simulink model "ros2_symulink_ettorone_mujoco"  (R2025b)
settings: Solver=ode4  StartTime=0.0  StopTime=inf  FixedStep=0.002  RelTol=1e-3
libraries: slpidlib x12, ros2lib x5
settings Model: Creator=ema  LastModifiedBy=ema

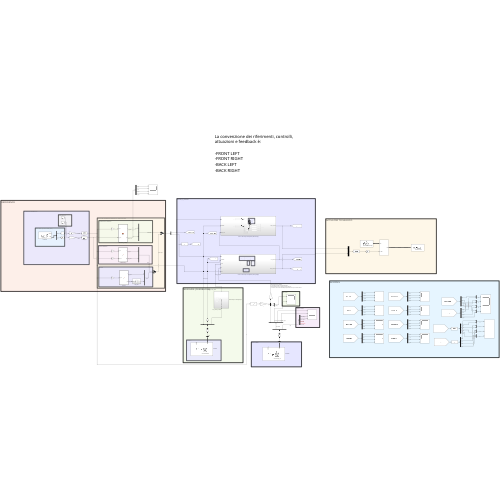
[thumbnail: Simulink's stored preview of the top-level diagram]
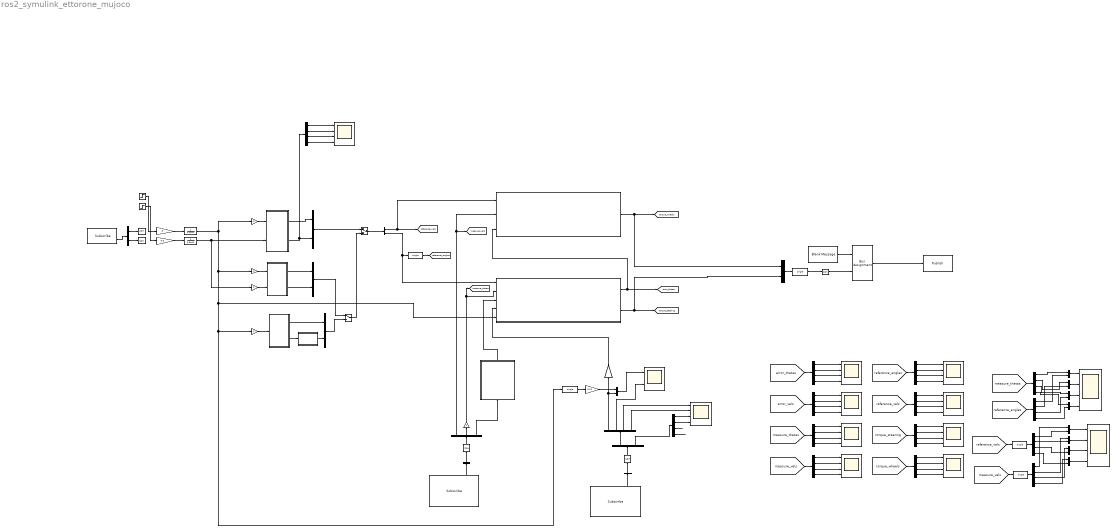
== system ros2_symulink_ettorone_mujoco ==
  note: La convenzione dei riferimenti, controlli, attuazioni e feedback è:
      |
      | -FRONT LEFT
      | -FRONT RIGHT
      | -BACK LEFT
      | -BACK RIGHT
  note: WHEELS SLIPS
  note: body_twist
  note: BODY FRAME
  note: WHEELS
  note: LOW LEVEL REFERENCE GENERATOR / MODE CONTROL
  note: SPIN360
  note: ROS2 INPUT (JOYSTIC CMD_VEL)
  note: const reference
  note: SCOPES
  note: MOTORS_&_CONTROL
  note: MEASURE (FEEDBACKS)
  note: ACTUATOR TO MUJOCO
  note: REFERENCE
  note: REFERENCE GENERATOR
  note: ACKERMANN STEERING
  note: CRAB STEERING
  Blank Message : ros2lib/Blank Message  messageClass=Message  entityType=interfaces/Float32Array8  messageType=interfaces/Float32Array8  SampleTime=0.002
  Bus Assignment : BusAssignment  AssignedSignals=data
  Bus Selector : BusSelector  OutputSignals=data
  Bus Selector1 : BusSelector  OutputSignals=linear.x,angular.z
  Bus Selector2 : BusSelector  OutputSignals=data
  Crab steering : MATLAB Function  TreatAsAtomicUnit=on
  Data Type Conversion{1..5} (5 alike) : DataTypeConversion  OutDataTypeStr=single  SaturateOnIntegerOverflow=off  RndMeth=Floor
  Demux1 : Demux  Outputs=3
  Demux{2..4,6..13,16..19} (15 alike) : Demux
  Demux15 : Demux  Outputs=2
  Demux5 : Demux  Outputs=2
  Gain : Gain
  Gain1 : Gain  Gain=8
  Gain2 : Gain  Gain=0.5
  Gain3 : Gain  Gain=1/0.12
  Gain5 : Gain  Gain=-1
  Gain6 : Gain
  Gain7 : Gain  Gain=-1
  Gain8 : Gain  Gain=-1
  Manual Switch : ManualSwitch
  Manual Switch1 : ManualSwitch
  Mux{,1..7,9..13} (13 alike) : Mux  Inputs=2
  Publish : ros2lib/Publish  topicSource=Specify your own  topic=/ettorone/actuator  messageType=interfaces/Float32Array8  QOSHistory=Keep last  QOSDepth=10  QOSReliability=Reliable  QOSDurability=Volatile  QOSDeadline=Inf  QOSLifespan=Inf  QOSLiveliness=Automatic  QOSLeaseDuration=Inf  QOSAvoidROSNamespaceConventions=off
  Scope{1..10,12..13} (12 alike) : Scope  NumInputPorts=4
      Scope1 settings: ActiveDisplayYMinimum=-24.08971523267201  ActiveDisplayYMaximum=2.6766350258524776
      Scope10 settings: ActiveDisplayString=4  ActiveDisplayYMinimum=-0.352103733781405  ActiveDisplayYMaximum=0.039646837980399134  DataLoggingVariableName=ScopeData10
      Scope12 settings: ActiveDisplayString=4  ActiveDisplayYMinimum=-12.276754975318909  ActiveDisplayYMaximum=1.3640838861465452  DataLoggingVariableName=ScopeData13
      Scope13 settings: ActiveDisplayYMinimum=-0.22020444087684155  ActiveDisplayYMaximum=0.25354055874049664  DataLoggingVariableName=ScopeData12
      Scope2 settings: ActiveDisplayYMinimum=-24.08971523267201  ActiveDisplayYMaximum=2.6766350258524776  DataLoggingVariableName=ScopeData3
      Scope3 settings: ActiveDisplayYMinimum=-24.08971523267201  ActiveDisplayYMaximum=2.6766350258524776
      Scope4 settings: ActiveDisplayYMinimum=-24.08971523267201  ActiveDisplayYMaximum=2.6766350258524776  DataLoggingVariableName=ScopeData2
      Scope5 settings: ActiveDisplayYMinimum=-24.08971523267201  ActiveDisplayYMaximum=2.6766350258524776  DataLoggingVariableName=ScopeData4
      Scope6 settings: ActiveDisplayYMinimum=-24.08971523267201  ActiveDisplayYMaximum=2.6766350258524776  DataLoggingVariableName=ScopeData5
      Scope7 settings: ActiveDisplayYMinimum=-24.08971523267201  ActiveDisplayYMaximum=2.6766350258524776  DataLoggingVariableName=ScopeData6
      Scope8 settings: ActiveDisplayYMinimum=-24.08971523267201  ActiveDisplayYMaximum=2.6766350258524776  DataLoggingVariableName=ScopeData7
      Scope9 settings: ActiveDisplayYMinimum=-0.038596316224778507  ActiveDisplayYMaximum=0.3473668460230066  DataLoggingVariableName=ScopeData8
  Scope11 : Scope  NumInputPorts=2
      settings: ActiveDisplayYMinimum=-0.10174171955077324  ActiveDisplayYMaximum=0.915423120426567  DataLoggingVariableName=ScopeData11
  Step : Step  Time=0  SampleTime=0
  Step1 : Step  Time=10  After=0.5  SampleTime=0
  Wheel Torque to Steering Torque : Subsystem
  Zero-Order Hold{,1..4} (5 alike) : ZeroOrderHold  SampleTime=0.002
  ackermann_geometry : MATLAB Function  TreatAsAtomicUnit=on
  control + motor torque linear dynamic (steering angles) : Subsystem
  control + motor torque linear dynamic (wheel velocity) : Subsystem
  feedback : ros2lib/Subscribe  topicSource=Specify your own  topic=/ettorone/feedback  messageType=interfaces/Float32Array12  sampleTime=0.002  QOSHistory=Keep last  QOSDepth=10  QOSReliability=Best effort  QOSDurability=Volatile  QOSDeadline=Inf  QOSLifespan=Inf  QOSLiveliness=Automatic  QOSLeaseDuration=Inf  QOSAvoidROSNamespaceConventions=off
  feedback1 : ros2lib/Subscribe  topicSource=Specify your own  topic=/joy/cmd_vel  messageType=geometry_msgs/Twist  sampleTime=0.002  QOSHistory=Keep last  QOSDepth=10  QOSReliability=Best effort  QOSDurability=Volatile  QOSDeadline=Inf  QOSLifespan=Inf  QOSLiveliness=Automatic  QOSLeaseDuration=Inf  QOSAvoidROSNamespaceConventions=off
  feedback2 : ros2lib/Subscribe  topicSource=Specify your own  topic=/ettorone/body_vel  messageType=interfaces/Float32Array8  sampleTime=0.002  QOSHistory=Keep last  QOSDepth=10  QOSReliability=Best effort  QOSDurability=Volatile  QOSDeadline=Inf  QOSLifespan=Inf  QOSLiveliness=Automatic  QOSLeaseDuration=Inf  QOSAvoidROSNamespaceConventions=off
  filters_a : TransferFcn  Denominator=[0.5 1]
  filters_v : TransferFcn  Denominator=[0.1 1]
  r : Gain  Gain=0.12
  spin mod : MATLAB Function  TreatAsAtomicUnit=on
  spin_filters : Subsystem
  tag scope: error_thetas=global, measure_thetas=global, measure_vels=global, reference_angles=global, reference_vels=global, torque_steering=global, torque_wheels=global
  wires:
  Blank Message/1 -> Bus Assignment/1
  Bus Assignment/1 -> Publish/1
  Zero-Order Hold/1 -> Demux1/1
  control + motor torque linear dynamic (wheel velocity)/1(Torque_wheels) -> [torque_wheels], Mux/1
  Demux1/1 -> control + motor torque linear dynamic (wheel velocity)/2(feedback), [measure_vels]  "wheels_vels"
  Demux1/2 -> Gain/1
  feedback/2 -> Bus Selector/1
  Bus Selector/1 -> Zero-Order Hold/1  "<data>"
  Zero-Order Hold2/1 -> Bus Assignment/2
  Mux/1 -> Data Type Conversion1/1
  Data Type Conversion1/1 -> Zero-Order Hold2/1
  Gain/1 -> [measure_thetas], control + motor torque linear dynamic (steering angles)/2(feedback)  "wheels_steering_angles"
  control + motor torque linear dynamic (steering angles)/2(Torque_steering) -> [torque_steering], Mux/2
  Bus Selector1/1 -> Zero-Order Hold1/1  "<x>"
  feedback1/2 -> Bus Selector1/1
  Bus Selector1/2 -> Zero-Order Hold3/1  "<z>"
  Crab steering/1(v) -> Mux3/1  "v_k_des"
  Crab steering/2(phi) -> Mux3/2  "phi_k_des"
  ackermann_geometry/2(phi) -> Demux11/1, Mux1/2  "phi_k_des"
  Manual Switch/1 -> Demux5/1
  Mux1/1 -> Manual Switch/1  "ackermann"
  ackermann_geometry/1(v) -> Mux1/1  "v_k_des"
  Demux5/1 -> [reference_vels], control + motor torque linear dynamic (wheel velocity)/1(ref)
  filters_a/1 -> ackermann_geometry/2(phi_des), Gain6/1
  Gain5/1 -> Crab steering/1(v_des)
  Gain6/1 -> Crab steering/2(phi_des)
  Gain7/1 -> ackermann_geometry/1(v_des)
  Demux1/3 -> Wheel Torque to Steering Torque/1(torque_whhels_feedback)  "torque_wheels_feedback"
  Wheel Torque to Steering Torque/1(Out1) -> control + motor torque linear dynamic (steering angles)/3(torch)  "torque_projected"
  control + motor torque linear dynamic (steering angles)/1(error_steering) -> [error_thetas], control + motor torque linear dynamic (wheel velocity)/3(theta_error)
  [error_thetas] -> Demux2/1
  [error_vels] -> Demux3/1
  Demux2/1 -> Scope6/1  "e_th_fl"
  Demux2/2 -> Scope6/2  "e_th_fr"
  Demux2/3 -> Scope6/3  "e_th_bl"
  Demux2/4 -> Scope6/4  "e_th_br"
  Demux3/1 -> Scope5/1  "e_v_fl"
  Demux3/2 -> Scope5/2  "e_v_fr"
  Demux3/3 -> Scope5/3  "e_v_bl"
  Demux3/4 -> Scope5/4  "e_v_br"
  Demux4/2 -> Scope2/2  "th_fr"
  Demux6/4 -> Scope1/4  "v_br"
  Demux6/2 -> Scope1/2  "v_fr"
  [measure_thetas] -> Demux4/1
  Demux6/3 -> Scope1/3  "v_bl"
  [measure_vels] -> Demux6/1
  Demux4/1 -> Scope2/1  "th_fl"
  Demux6/1 -> Scope1/1  "v_fl"
  Demux4/3 -> Scope2/3  "th_bl"
  Demux4/4 -> Scope2/4  "th_br"
  Demux7/2 -> Scope3/2  "r_th_fr"
  Demux8/4 -> Scope4/4  "r_v_br"
  Demux8/2 -> Scope4/2  "r_v_fr"
  [reference_angles] -> Demux7/1
  Demux8/3 -> Scope4/3  "r_v_bl"
  [reference_vels] -> Demux8/1
  Demux7/1 -> Scope3/1  "r_th_fl"
  Demux8/1 -> Scope4/1  "r_v_fl"
  Demux7/3 -> Scope3/3  "r_th_bl"
  Demux7/4 -> Scope3/4  "r_th_br"
  Demux9/4 -> Scope7/4  "t_th_br"
  [torque_steering] -> Demux9/1
  [torque_wheels] -> Demux10/1
  Demux10/4 -> Scope8/4  "t_v_br"
  Demux10/2 -> Scope8/2  "t_v_fr"
  Demux10/3 -> Scope8/3  "t_v_bl"
  Demux9/3 -> Scope7/3  "t_th_bl"
  Demux9/1 -> Scope7/1  "t_th_fl"
  Demux10/1 -> Scope8/1  "t_v_fl"
  Demux9/2 -> Scope7/2  "t_th_fr"
  Demux11/4 -> Scope9/4  "r_th_br"
  Demux11/3 -> Scope9/3  "r_th_bl"
  Demux11/1 -> Scope9/1  "r_th_fl"
  Demux11/2 -> Scope9/2  "r_th_fr"
  [reference_angles] -> Demux13/1
  Mux2/1 -> Scope10/1  "fl"
  Mux4/1 -> Scope10/2  "fr"
  Mux5/1 -> Scope10/3  "bl"
  Demux13/1 -> Mux2/2  "r_th_fl"
  Demux13/2 -> Mux4/2  "r_th_fr"
  Demux13/3 -> Mux5/2  "r_th_bl"
  Demux13/4 -> Mux6/2  "r_th_br"
  Mux6/1 -> Scope10/4  "br"
  Demux12/2 -> Mux4/1  "v_fr"
  [measure_thetas] -> Demux12/1
  Demux12/3 -> Mux5/1  "v_bl"
  Demux12/1 -> Mux2/1  "v_fl"
  Demux12/4 -> Mux6/1  "v_br"
  Data Type Conversion2/1 -> [reference_angles]
  Demux5/2 -> control + motor torque linear dynamic (steering angles)/1(ref), Data Type Conversion2/1
  spin mod/1(v) -> Mux7/1  "v_k_des"
  Mux3/1 -> Manual Switch1/1  "grab"
  Mux7/1 -> Manual Switch1/2  "spin"
  Manual Switch1/1 -> Manual Switch/2  "grab or spin"
  feedback2/2 -> Bus Selector2/1
  Zero-Order Hold4/1 -> Demux15/1
  Bus Selector2/1 -> Zero-Order Hold4/1  "<data>"
  Demux16/2 -> Scope11/2  "yaw_rate"
  Demux16/1 -> Gain3/1, Mux13/2  "vx"
  Demux15/1 -> Demux16/1  "vels & slips"
  Gain1/1 -> filters_v/1  "velocities"
  Gain2/1 -> filters_a/1  "angles"
  Gain3/1 -> control + motor torque linear dynamic (steering angles)/4(vx)  "volendo questo si puo cambiare è un termine che prende la velocità longitudinale nel body frame del rover è lo divide per il raggio delle ruote. cosi da avere due velocità confrontabili per il gain dinamico del FF per il sistema di sterzo"
  [reference_vels] -> Data Type Conversion5/1
  Mux12/1 -> Scope12/4  "br"
  Mux10/1 -> Scope12/2  "fr"
  Mux11/1 -> Scope12/3  "bl"
  Mux9/1 -> Scope12/1  "fl"
  [measure_vels] -> Data Type Conversion4/1
  Mux13/1 -> Scope11/1  "v_long"
  Data Type Conversion3/1 -> r/1
  Data Type Conversion4/1 -> Demux18/1
  Data Type Conversion5/1 -> Demux17/1
  Demux15/2 -> Demux19/1  "slip"
  Demux16/3 -> Scope13/1  "angle_slip_fl"
  Demux16/4 -> Scope13/2  "angle_slip_fr"
  Demux19/1 -> Scope13/3  "angle_slip_bl"
  Demux19/2 -> Scope13/4  "angle_slip_br"
  filters_v/1 -> Data Type Conversion3/1, Gain8/1, control + motor torque linear dynamic (steering angles)/5(vref), Gain5/1, Gain7/1  "w"
  r/1 -> Mux13/1  "v_long_ref"
  Demux17/1 -> Mux9/2  "r_v_fl"
  Demux17/2 -> Mux10/2  "r_v_fr"
  Demux17/3 -> Mux11/2  "r_v_bl"
  Demux17/4 -> Mux12/2  "r_v_br"
  Demux18/1 -> Mux9/1  "v_fl"
  Demux18/2 -> Mux10/1  "v_fr"
  Demux18/3 -> Mux11/1  "v_bl"
  Demux18/4 -> Mux12/1  "v_br"
  Step/1 -> Gain1/1  "rotational speed ref"
  Step1/1 -> Gain2/1
  Gain8/1 -> spin mod/1(v_des)
  spin mod/2(phi) -> spin_filters/1(phi_k_des)  "phi_k_des"
  spin_filters/1(Out1) -> Mux7/2
  Demux19/3 -> ?  "non usato"
  Demux19/4 -> ?  "non usato"

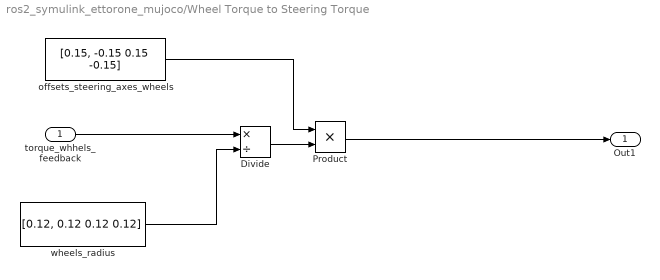
== system ros2_symulink_ettorone_mujoco/Wheel Torque to Steering Torque ==
  torque_whhels_feedback : Inport
  Divide : Product  Inputs=*/
  Product : Product
  offsets_steering_axes_wheels : Constant  Value=[0.15, -0.15 0.15 -0.15]
  wheels_radius : Constant  Value=[0.12, 0.12 0.12 0.12]
  Out1 : Outport
  wires:
  wheels_radius/1 -> Divide/2
  Divide/1 -> Product/2
  offsets_steering_axes_wheels/1 -> Product/1
  torque_whhels_feedback/1 -> Divide/1
  Product/1 -> Out1/1

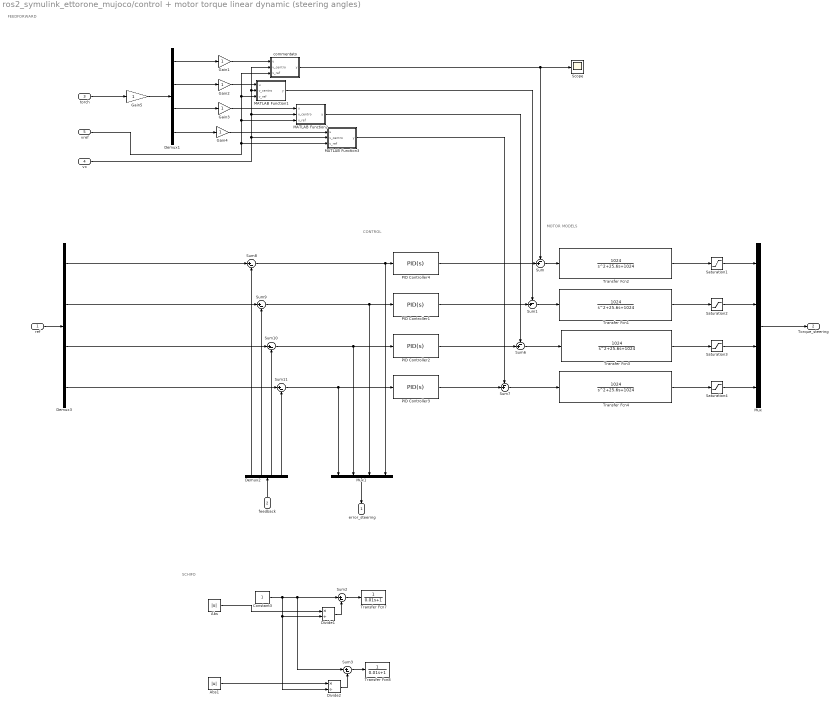
== system ros2_symulink_ettorone_mujoco/control + motor torque linear dynamic (steering angles) ==
  note: SCHIFO
  note: MOTOR MODELS
  note: CONTROL
  note: FEEDFORWARD
  ref : Inport
  feedback : Inport  Port=2
  torch : Inport  Port=3
  vx : Inport  Port=4
  vref : Inport  Port=5
  Abs : Abs  SaturateOnIntegerOverflow=off
  Abs1 : Abs  SaturateOnIntegerOverflow=off
  Constant3 : Constant
  Demux1 : Demux
  Demux2 : Demux
  Demux3 : Demux
  Divide1 : Product  Inputs=*/
  Divide2 : Product  Inputs=*/
  Gain{1..5} (5 alike) : Gain
  MATLAB Function1 : MATLAB Function  TreatAsAtomicUnit=on
  MATLAB Function2 : MATLAB Function  TreatAsAtomicUnit=on
  MATLAB Function3 : MATLAB Function  TreatAsAtomicUnit=on
  Mux : Mux
  Mux1 : Mux
  PID Controller1 : slpidlib/PID Controller  Controller=PID  Form=Parallel  TimeDomain=Continuous-time  UseExternalTs=off  SampleTime=-1  IntegratorMethod=Forward Euler  FilterMethod=Forward Euler  ControllerParametersSource=internal  P=30  I=4  UseKiTs=off  D=0  UseExternalDerivativeSource=off  N=100  UseFilter=on  TunerSelectOption=Transfer Function Based (PID Tuner App)  InitialConditionSource=internal  InitialConditionForIntegrator=0  InitialConditionForFilter=0  DifferentiatorICPrevScaledInput=0  ExternalReset=none  TrackingMode=off  Kt=1  LimitOutput=on  SatLimitsSource=internal  UpperSaturationLimit=25  LowerSaturationLimit=-25  LinearizeAsGain=on  AntiWindupMode=back-calculation  Kb=1  LimitIntegrator=off  UpperIntegratorSaturationLimit=inf  LowerIntegratorSaturationLimit=-inf  POutMin=[]  POutMax=[]  IOutMin=[]  IOutMax=[]  DOutMin=[]  DOutMax=[]  NOutMin=[]  NOutMax=[]  SumOutMin=[]  SumOutMax=[]  SaturationOutMin=[]  SaturationOutMax=[]  PParamMin=[]  PParamMax=[]  IParamMin=[]  IParamMax=[]  DParamMin=[]  DParamMax=[]  NParamMin=[]  NParamMax=[]  KbParamMin=[]  KbParamMax=[]  KtParamMin=[]  KtParamMax=[]  KbOutMin=[]  KbOutMax=[]  KtOutMin=[]  KtOutMax=[]  IntegratorOutMin=[]  IntegratorOutMax=[]  FilterOutMin=[]  FilterOutMax=[]  SumI1OutMin=[]  SumI1OutMax=[]  SumI2OutMin=[]  SumI2OutMax=[]  SumI3OutMin=[]  SumI3OutMax=[]  SumI4OutMin=[]  SumI4OutMax=[]  SumDOutMin=[]  SumDOutMax=[]  DifferentiatorOutMin=[]  DifferentiatorOutMax=[]  FilterDiffOutCoefMin=[]  FilterDiffOutCoefMax=[]  ReciprocalOutMin=[]  ReciprocalOutMax=[]  SumDenOutMin=[]  SumDenOutMax=[]  SumNumOutMin=[]  SumNumOutMax=[]  DivideOutMin=[]  DivideOutMax=[]  UdiffTsProdOutMin=[]  UdiffTsProdOutMax=[]  NTsProdOutMin=[]  NTsProdOutMax=[]  UintegralTsProdOutMin=[]  UintegralTsProdOutMax=[]  UngainTsProdOutMin=[]  UngainTsProdOutMax=[]  ClampingZeroOutDataTypeStr=Inherit: Inherit via back propagation  ClampingZeroOutMin=[]  ClampingZeroOutMax=[]  FilterDenConstantOutDataTypeStr=Inherit: Inherit via back propagation  FilterDenConstantOutMin=[]  FilterDenConstantOutMax=[]  PCopyOutDataTypeStr=Inherit: Inherit via back propagation  PCopyOutMin=[]  PCopyOutMax=[]  NCopyOutDataTypeStr=Inherit: Inherit via back propagation  NCopyOutMin=[]  NCopyOutMax=[]  IntegratorContinuousStateAttributes=''  IntegratorStateMustResolveToSignalObject=off  IntegratorRTWStateStorageClass=Auto  FilterContinuousStateAttributes=''  FilterStateMustResolveToSignalObject=off  FilterRTWStateStorageClass=Auto  ParallelPVariant=InternalParameters  IdealPVariant=Disabled  IVariant=InternalParameters  DVariant=InternalParameters  IntegratorVariant=Continuous  SatVariant=Enabled  AWVariant=BackCalculation  PCopyVariant=Disabled  TRVariant=Disabled  FdbkBlocksVariant=Forward  IdealPFdbkVariant=Disabled  SatFdbkVariant=Disabled  DerivativeFilterVariant=ContFilter  NVariant=InternalParameters  NCopyVariant=Disabled  FilterICVariant=InternalICsFilter  IntegratorICVariant=InternalICs  ExternalResetVariant=Disabled  TRSumVariant=Passthrough  SumFdbkVariant=Disabled  SumVariant=Sum_PID  TsampFilterVariant=InternalTs  TsampNgainVariant=Passthrough  TsampIntegralVariant=Disabled_SignalSpec  ExternalSaturationOutDataTypeStr=Inherit: Same as second input  DerivativeSourceVariant=ErrorSignal  PreIntVariant=InternalPreInt
  PID Controller2 : slpidlib/PID Controller  Controller=PID  Form=Parallel  TimeDomain=Continuous-time  UseExternalTs=off  SampleTime=-1  IntegratorMethod=Forward Euler  FilterMethod=Forward Euler  ControllerParametersSource=internal  P=30  I=4  UseKiTs=off  D=3  UseExternalDerivativeSource=off  N=10  UseFilter=on  TunerSelectOption=Transfer Function Based (PID Tuner App)  InitialConditionSource=internal  InitialConditionForIntegrator=0  InitialConditionForFilter=0  DifferentiatorICPrevScaledInput=0  ExternalReset=none  TrackingMode=off  Kt=1  LimitOutput=on  SatLimitsSource=internal  UpperSaturationLimit=25  LowerSaturationLimit=-25  LinearizeAsGain=on  AntiWindupMode=back-calculation  Kb=1  LimitIntegrator=off  UpperIntegratorSaturationLimit=inf  LowerIntegratorSaturationLimit=-inf  POutMin=[]  POutMax=[]  IOutMin=[]  IOutMax=[]  DOutMin=[]  DOutMax=[]  NOutMin=[]  NOutMax=[]  SumOutMin=[]  SumOutMax=[]  SaturationOutMin=[]  SaturationOutMax=[]  PParamMin=[]  PParamMax=[]  IParamMin=[]  IParamMax=[]  DParamMin=[]  DParamMax=[]  NParamMin=[]  NParamMax=[]  KbParamMin=[]  KbParamMax=[]  KtParamMin=[]  KtParamMax=[]  KbOutMin=[]  KbOutMax=[]  KtOutMin=[]  KtOutMax=[]  IntegratorOutMin=[]  IntegratorOutMax=[]  FilterOutMin=[]  FilterOutMax=[]  SumI1OutMin=[]  SumI1OutMax=[]  SumI2OutMin=[]  SumI2OutMax=[]  SumI3OutMin=[]  SumI3OutMax=[]  SumI4OutMin=[]  SumI4OutMax=[]  SumDOutMin=[]  SumDOutMax=[]  DifferentiatorOutMin=[]  DifferentiatorOutMax=[]  FilterDiffOutCoefMin=[]  FilterDiffOutCoefMax=[]  ReciprocalOutMin=[]  ReciprocalOutMax=[]  SumDenOutMin=[]  SumDenOutMax=[]  SumNumOutMin=[]  SumNumOutMax=[]  DivideOutMin=[]  DivideOutMax=[]  UdiffTsProdOutMin=[]  UdiffTsProdOutMax=[]  NTsProdOutMin=[]  NTsProdOutMax=[]  UintegralTsProdOutMin=[]  UintegralTsProdOutMax=[]  UngainTsProdOutMin=[]  UngainTsProdOutMax=[]  ClampingZeroOutDataTypeStr=Inherit: Inherit via back propagation  ClampingZeroOutMin=[]  ClampingZeroOutMax=[]  FilterDenConstantOutDataTypeStr=Inherit: Inherit via back propagation  FilterDenConstantOutMin=[]  FilterDenConstantOutMax=[]  PCopyOutDataTypeStr=Inherit: Inherit via back propagation  PCopyOutMin=[]  PCopyOutMax=[]  NCopyOutDataTypeStr=Inherit: Inherit via back propagation  NCopyOutMin=[]  NCopyOutMax=[]  IntegratorContinuousStateAttributes=''  IntegratorStateMustResolveToSignalObject=off  IntegratorRTWStateStorageClass=Auto  FilterContinuousStateAttributes=''  FilterStateMustResolveToSignalObject=off  FilterRTWStateStorageClass=Auto  ParallelPVariant=InternalParameters  IdealPVariant=Disabled  IVariant=InternalParameters  DVariant=InternalParameters  IntegratorVariant=Continuous  SatVariant=Enabled  AWVariant=BackCalculation  PCopyVariant=Disabled  TRVariant=Disabled  FdbkBlocksVariant=Forward  IdealPFdbkVariant=Disabled  SatFdbkVariant=Disabled  DerivativeFilterVariant=ContFilter  NVariant=InternalParameters  NCopyVariant=Disabled  FilterICVariant=InternalICsFilter  IntegratorICVariant=InternalICs  ExternalResetVariant=Disabled  TRSumVariant=Passthrough  SumFdbkVariant=Disabled  SumVariant=Sum_PID  TsampFilterVariant=InternalTs  TsampNgainVariant=Passthrough  TsampIntegralVariant=Disabled_SignalSpec  ExternalSaturationOutDataTypeStr=Inherit: Same as second input  DerivativeSourceVariant=ErrorSignal  PreIntVariant=InternalPreInt
  PID Controller3 : slpidlib/PID Controller  Controller=PID  Form=Parallel  TimeDomain=Continuous-time  UseExternalTs=off  SampleTime=-1  IntegratorMethod=Forward Euler  FilterMethod=Forward Euler  ControllerParametersSource=internal  P=30  I=4  UseKiTs=off  D=2  UseExternalDerivativeSource=off  N=10  UseFilter=on  TunerSelectOption=Transfer Function Based (PID Tuner App)  InitialConditionSource=internal  InitialConditionForIntegrator=0  InitialConditionForFilter=0  DifferentiatorICPrevScaledInput=0  ExternalReset=none  TrackingMode=off  Kt=1  LimitOutput=on  SatLimitsSource=internal  UpperSaturationLimit=25  LowerSaturationLimit=-25  LinearizeAsGain=on  AntiWindupMode=back-calculation  Kb=1  LimitIntegrator=off  UpperIntegratorSaturationLimit=inf  LowerIntegratorSaturationLimit=-inf  POutMin=[]  POutMax=[]  IOutMin=[]  IOutMax=[]  DOutMin=[]  DOutMax=[]  NOutMin=[]  NOutMax=[]  SumOutMin=[]  SumOutMax=[]  SaturationOutMin=[]  SaturationOutMax=[]  PParamMin=[]  PParamMax=[]  IParamMin=[]  IParamMax=[]  DParamMin=[]  DParamMax=[]  NParamMin=[]  NParamMax=[]  KbParamMin=[]  KbParamMax=[]  KtParamMin=[]  KtParamMax=[]  KbOutMin=[]  KbOutMax=[]  KtOutMin=[]  KtOutMax=[]  IntegratorOutMin=[]  IntegratorOutMax=[]  FilterOutMin=[]  FilterOutMax=[]  SumI1OutMin=[]  SumI1OutMax=[]  SumI2OutMin=[]  SumI2OutMax=[]  SumI3OutMin=[]  SumI3OutMax=[]  SumI4OutMin=[]  SumI4OutMax=[]  SumDOutMin=[]  SumDOutMax=[]  DifferentiatorOutMin=[]  DifferentiatorOutMax=[]  FilterDiffOutCoefMin=[]  FilterDiffOutCoefMax=[]  ReciprocalOutMin=[]  ReciprocalOutMax=[]  SumDenOutMin=[]  SumDenOutMax=[]  SumNumOutMin=[]  SumNumOutMax=[]  DivideOutMin=[]  DivideOutMax=[]  UdiffTsProdOutMin=[]  UdiffTsProdOutMax=[]  NTsProdOutMin=[]  NTsProdOutMax=[]  UintegralTsProdOutMin=[]  UintegralTsProdOutMax=[]  UngainTsProdOutMin=[]  UngainTsProdOutMax=[]  ClampingZeroOutDataTypeStr=Inherit: Inherit via back propagation  ClampingZeroOutMin=[]  ClampingZeroOutMax=[]  FilterDenConstantOutDataTypeStr=Inherit: Inherit via back propagation  FilterDenConstantOutMin=[]  FilterDenConstantOutMax=[]  PCopyOutDataTypeStr=Inherit: Inherit via back propagation  PCopyOutMin=[]  PCopyOutMax=[]  NCopyOutDataTypeStr=Inherit: Inherit via back propagation  NCopyOutMin=[]  NCopyOutMax=[]  IntegratorContinuousStateAttributes=''  IntegratorStateMustResolveToSignalObject=off  IntegratorRTWStateStorageClass=Auto  FilterContinuousStateAttributes=''  FilterStateMustResolveToSignalObject=off  FilterRTWStateStorageClass=Auto  ParallelPVariant=InternalParameters  IdealPVariant=Disabled  IVariant=InternalParameters  DVariant=InternalParameters  IntegratorVariant=Continuous  SatVariant=Enabled  AWVariant=BackCalculation  PCopyVariant=Disabled  TRVariant=Disabled  FdbkBlocksVariant=Forward  IdealPFdbkVariant=Disabled  SatFdbkVariant=Disabled  DerivativeFilterVariant=ContFilter  NVariant=InternalParameters  NCopyVariant=Disabled  FilterICVariant=InternalICsFilter  IntegratorICVariant=InternalICs  ExternalResetVariant=Disabled  TRSumVariant=Passthrough  SumFdbkVariant=Disabled  SumVariant=Sum_PID  TsampFilterVariant=InternalTs  TsampNgainVariant=Passthrough  TsampIntegralVariant=Disabled_SignalSpec  ExternalSaturationOutDataTypeStr=Inherit: Same as second input  DerivativeSourceVariant=ErrorSignal  PreIntVariant=InternalPreInt
  PID Controller4 : slpidlib/PID Controller  Controller=PID  Form=Parallel  TimeDomain=Continuous-time  UseExternalTs=off  SampleTime=-1  IntegratorMethod=Forward Euler  FilterMethod=Forward Euler  ControllerParametersSource=internal  P=30  I=4  UseKiTs=off  D=0  UseExternalDerivativeSource=off  N=100  UseFilter=on  TunerSelectOption=Transfer Function Based (PID Tuner App)  InitialConditionSource=internal  InitialConditionForIntegrator=0  InitialConditionForFilter=0  DifferentiatorICPrevScaledInput=0  ExternalReset=none  TrackingMode=off  Kt=1  LimitOutput=on  SatLimitsSource=internal  UpperSaturationLimit=25  LowerSaturationLimit=-25  LinearizeAsGain=on  AntiWindupMode=back-calculation  Kb=1  LimitIntegrator=off  UpperIntegratorSaturationLimit=inf  LowerIntegratorSaturationLimit=-inf  POutMin=[]  POutMax=[]  IOutMin=[]  IOutMax=[]  DOutMin=[]  DOutMax=[]  NOutMin=[]  NOutMax=[]  SumOutMin=[]  SumOutMax=[]  SaturationOutMin=[]  SaturationOutMax=[]  PParamMin=[]  PParamMax=[]  IParamMin=[]  IParamMax=[]  DParamMin=[]  DParamMax=[]  NParamMin=[]  NParamMax=[]  KbParamMin=[]  KbParamMax=[]  KtParamMin=[]  KtParamMax=[]  KbOutMin=[]  KbOutMax=[]  KtOutMin=[]  KtOutMax=[]  IntegratorOutMin=[]  IntegratorOutMax=[]  FilterOutMin=[]  FilterOutMax=[]  SumI1OutMin=[]  SumI1OutMax=[]  SumI2OutMin=[]  SumI2OutMax=[]  SumI3OutMin=[]  SumI3OutMax=[]  SumI4OutMin=[]  SumI4OutMax=[]  SumDOutMin=[]  SumDOutMax=[]  DifferentiatorOutMin=[]  DifferentiatorOutMax=[]  FilterDiffOutCoefMin=[]  FilterDiffOutCoefMax=[]  ReciprocalOutMin=[]  ReciprocalOutMax=[]  SumDenOutMin=[]  SumDenOutMax=[]  SumNumOutMin=[]  SumNumOutMax=[]  DivideOutMin=[]  DivideOutMax=[]  UdiffTsProdOutMin=[]  UdiffTsProdOutMax=[]  NTsProdOutMin=[]  NTsProdOutMax=[]  UintegralTsProdOutMin=[]  UintegralTsProdOutMax=[]  UngainTsProdOutMin=[]  UngainTsProdOutMax=[]  ClampingZeroOutDataTypeStr=Inherit: Inherit via back propagation  ClampingZeroOutMin=[]  ClampingZeroOutMax=[]  FilterDenConstantOutDataTypeStr=Inherit: Inherit via back propagation  FilterDenConstantOutMin=[]  FilterDenConstantOutMax=[]  PCopyOutDataTypeStr=Inherit: Inherit via back propagation  PCopyOutMin=[]  PCopyOutMax=[]  NCopyOutDataTypeStr=Inherit: Inherit via back propagation  NCopyOutMin=[]  NCopyOutMax=[]  IntegratorContinuousStateAttributes=''  IntegratorStateMustResolveToSignalObject=off  IntegratorRTWStateStorageClass=Auto  FilterContinuousStateAttributes=''  FilterStateMustResolveToSignalObject=off  FilterRTWStateStorageClass=Auto  ParallelPVariant=InternalParameters  IdealPVariant=Disabled  IVariant=InternalParameters  DVariant=InternalParameters  IntegratorVariant=Continuous  SatVariant=Enabled  AWVariant=BackCalculation  PCopyVariant=Disabled  TRVariant=Disabled  FdbkBlocksVariant=Forward  IdealPFdbkVariant=Disabled  SatFdbkVariant=Disabled  DerivativeFilterVariant=ContFilter  NVariant=InternalParameters  NCopyVariant=Disabled  FilterICVariant=InternalICsFilter  IntegratorICVariant=InternalICs  ExternalResetVariant=Disabled  TRSumVariant=Passthrough  SumFdbkVariant=Disabled  SumVariant=Sum_PID  TsampFilterVariant=InternalTs  TsampNgainVariant=Passthrough  TsampIntegralVariant=Disabled_SignalSpec  ExternalSaturationOutDataTypeStr=Inherit: Same as second input  DerivativeSourceVariant=ErrorSignal  PreIntVariant=InternalPreInt
  Saturation{1..4} (4 alike) : Saturate  UpperLimit=17  LowerLimit=-17
  Scope : Scope
      settings: ActiveDisplayYMinimum=-1  ActiveDisplayYMaximum=1  DataLoggingVariableName=ScopeData12
  Sum{,1,6..7} (4 alike) : Sum  Inputs=-+|
  Sum{2..3,8..11} (6 alike) : Sum  Inputs=|+-
  Transfer Fcn{1..4} (4 alike) : TransferFcn  Numerator=[1024]  Denominator="[1  25.6 1024]"
  Transfer Fcn7 : TransferFcn  Denominator=[0.01 1]
  Transfer Fcn8 : TransferFcn  Denominator=[0.01 1]
  commentato : MATLAB Function  TreatAsAtomicUnit=on
  error_steering : Outport
  Torque_steering : Outport  Port=2
  wires:
  Mux/1 -> Torque_steering/1
  feedback/1 -> Demux2/1
  Mux1/1 -> error_steering/1
  Transfer Fcn1/1 -> Saturation2/1
  Transfer Fcn2/1 -> Saturation1/1
  Transfer Fcn3/1 -> Saturation3/1
  Transfer Fcn4/1 -> Saturation4/1
  torch/1 -> Gain5/1
  Sum/1 -> Transfer Fcn2/1
  Sum7/1 -> Transfer Fcn4/1
  Sum6/1 -> Transfer Fcn3/1
  Sum1/1 -> Transfer Fcn1/1
  Demux1/1 -> Gain1/1
  Demux1/2 -> Gain2/1
  Demux1/3 -> Gain3/1
  Demux1/4 -> Gain4/1
  ref/1 -> Demux3/1
  PID Controller4/1 -> Sum/2
  PID Controller1/1 -> Sum1/2
  Demux2/1 -> Sum8/2
  Demux2/2 -> Sum9/2
  Demux2/3 -> Sum10/2
  Sum10/1 -> Mux1/2, PID Controller2/1
  Demux2/4 -> Sum11/2
  Sum9/1 -> Mux1/3, PID Controller1/1
  Sum8/1 -> Mux1/4, PID Controller4/1
  Divide1/1 -> Sum2/2
  Divide2/1 -> Sum3/2
  Constant3/1 -> Divide2/2, Divide1/2, Sum2/1, Sum3/1
  PID Controller2/1 -> Sum6/2
  PID Controller3/1 -> Sum7/2
  Sum2/1 -> Transfer Fcn7/1
  Sum3/1 -> Transfer Fcn8/1
  Gain5/1 -> Demux1/1
  Abs/1 -> Divide1/1
  Abs1/1 -> Divide2/1
  Saturation1/1 -> Mux/1
  Saturation2/1 -> Mux/2
  Saturation3/1 -> Mux/3
  Saturation4/1 -> Mux/4
  Demux3/3 -> Sum10/1
  Demux3/4 -> Sum11/1
  Gain1/1 -> commentato/1(u)
  Gain2/1 -> MATLAB Function1/1(u)
  Gain4/1 -> MATLAB Function3/1(u)
  Gain3/1 -> MATLAB Function2/1(u)
  vx/1 -> commentato/2(v_centro), MATLAB Function1/2(v_centro), MATLAB Function2/2(v_centro), MATLAB Function3/2(v_centro)
  vref/1 -> MATLAB Function3/3(v_ref), MATLAB Function2/3(v_ref), MATLAB Function1/3(v_ref), commentato/3(v_ref)
  commentato/1(y) -> Scope/1, Sum/1
  Sum11/1 -> PID Controller3/1, Mux1/1
  MATLAB Function3/1(y) -> Sum7/1
  MATLAB Function2/1(y) -> Sum6/1
  MATLAB Function1/1(y) -> Sum1/1
  Demux3/2 -> Sum9/1
  Demux3/1 -> Sum8/1

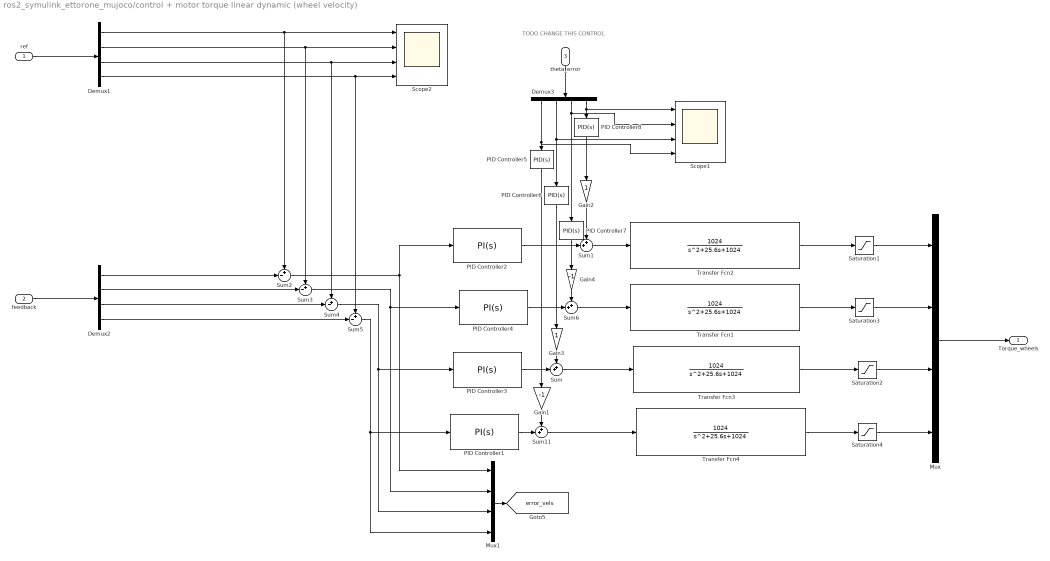
== system ros2_symulink_ettorone_mujoco/control + motor torque linear dynamic (wheel velocity) ==
  note: TODO CHANGE THIS CONTROL
  ref : Inport
  feedback : Inport  Port=2
  theta_error : Inport  Port=3
  Demux1 : Demux
  Demux2 : Demux
  Demux3 : Demux
  Gain1 : Gain  Gain=-1
  Gain2 : Gain
  Gain3 : Gain
  Gain4 : Gain  Gain=-1
  Mux : Mux
  Mux1 : Mux
  PID Controller{1..4} (4 alike) : slpidlib/PID Controller  Controller=PI  Form=Parallel  TimeDomain=Continuous-time  UseExternalTs=off  SampleTime=-1  IntegratorMethod=Forward Euler  FilterMethod=Forward Euler  ControllerParametersSource=internal  P=1  I=0.3  UseKiTs=off  D=0  UseExternalDerivativeSource=off  N=100  UseFilter=on  TunerSelectOption=Transfer Function Based (PID Tuner App)  InitialConditionSource=internal  InitialConditionForIntegrator=0  InitialConditionForFilter=0  DifferentiatorICPrevScaledInput=0  ExternalReset=none  TrackingMode=off  Kt=1  LimitOutput=off  SatLimitsSource=internal  UpperSaturationLimit=inf  LowerSaturationLimit=-inf  LinearizeAsGain=on  AntiWindupMode=none  Kb=1  LimitIntegrator=off  UpperIntegratorSaturationLimit=inf  LowerIntegratorSaturationLimit=-inf  POutMin=[]  POutMax=[]  IOutMin=[]  IOutMax=[]  DOutMin=[]  DOutMax=[]  NOutMin=[]  NOutMax=[]  SumOutMin=[]  SumOutMax=[]  SaturationOutMin=[]  SaturationOutMax=[]  PParamMin=[]  PParamMax=[]  IParamMin=[]  IParamMax=[]  DParamMin=[]  DParamMax=[]  NParamMin=[]  NParamMax=[]  KbParamMin=[]  KbParamMax=[]  KtParamMin=[]  KtParamMax=[]  KbOutMin=[]  KbOutMax=[]  KtOutMin=[]  KtOutMax=[]  IntegratorOutMin=[]  IntegratorOutMax=[]  FilterOutMin=[]  FilterOutMax=[]  SumI1OutMin=[]  SumI1OutMax=[]  SumI2OutMin=[]  SumI2OutMax=[]  SumI3OutMin=[]  SumI3OutMax=[]  SumI4OutMin=[]  SumI4OutMax=[]  SumDOutMin=[]  SumDOutMax=[]  DifferentiatorOutMin=[]  DifferentiatorOutMax=[]  FilterDiffOutCoefMin=[]  FilterDiffOutCoefMax=[]  ReciprocalOutMin=[]  ReciprocalOutMax=[]  SumDenOutMin=[]  SumDenOutMax=[]  SumNumOutMin=[]  SumNumOutMax=[]  DivideOutMin=[]  DivideOutMax=[]  UdiffTsProdOutMin=[]  UdiffTsProdOutMax=[]  NTsProdOutMin=[]  NTsProdOutMax=[]  UintegralTsProdOutMin=[]  UintegralTsProdOutMax=[]  UngainTsProdOutMin=[]  UngainTsProdOutMax=[]  ClampingZeroOutDataTypeStr=Inherit: Inherit via back propagation  ClampingZeroOutMin=[]  ClampingZeroOutMax=[]  FilterDenConstantOutDataTypeStr=Inherit: Inherit via back propagation  FilterDenConstantOutMin=[]  FilterDenConstantOutMax=[]  PCopyOutDataTypeStr=Inherit: Inherit via back propagation  PCopyOutMin=[]  PCopyOutMax=[]  NCopyOutDataTypeStr=Inherit: Inherit via back propagation  NCopyOutMin=[]  NCopyOutMax=[]  IntegratorContinuousStateAttributes=''  IntegratorStateMustResolveToSignalObject=off  IntegratorRTWStateStorageClass=Auto  FilterContinuousStateAttributes=''  FilterStateMustResolveToSignalObject=off  FilterRTWStateStorageClass=Auto  ParallelPVariant=InternalParameters  IdealPVariant=Disabled  IVariant=InternalParameters  DVariant=Disabled  IntegratorVariant=Continuous  SatVariant=Disabled  AWVariant=Passthrough  PCopyVariant=Disabled  TRVariant=Disabled  FdbkBlocksVariant=Forward  IdealPFdbkVariant=Disabled  SatFdbkVariant=Disabled  DerivativeFilterVariant=Disabled  NVariant=Disabled  NCopyVariant=Disabled_SignalSpec  FilterICVariant=Disabled  IntegratorICVariant=InternalICs  ExternalResetVariant=Disabled  TRSumVariant=Passthrough  SumFdbkVariant=Disabled  SumVariant=Sum_PI  TsampFilterVariant=InternalTs  TsampNgainVariant=Passthrough  TsampIntegralVariant=Disabled_SignalSpec  ExternalSaturationOutDataTypeStr=Inherit: Same as second input  DerivativeSourceVariant=Disabled  PreIntVariant=InternalPreInt
  PID Controller{5..8} (4 alike) : slpidlib/PID Controller  Controller=PID  Form=Parallel  TimeDomain=Continuous-time  UseExternalTs=off  SampleTime=-1  IntegratorMethod=Forward Euler  FilterMethod=Forward Euler  ControllerParametersSource=internal  P=10  I=0.5  UseKiTs=off  D=2.5  UseExternalDerivativeSource=off  N=10  UseFilter=on  TunerSelectOption=Transfer Function Based (PID Tuner App)  InitialConditionSource=internal  InitialConditionForIntegrator=0  InitialConditionForFilter=0  DifferentiatorICPrevScaledInput=0  ExternalReset=none  TrackingMode=off  Kt=1  LimitOutput=off  SatLimitsSource=internal  UpperSaturationLimit=inf  LowerSaturationLimit=-inf  LinearizeAsGain=on  AntiWindupMode=none  Kb=1  LimitIntegrator=off  UpperIntegratorSaturationLimit=inf  LowerIntegratorSaturationLimit=-inf  POutMin=[]  POutMax=[]  IOutMin=[]  IOutMax=[]  DOutMin=[]  DOutMax=[]  NOutMin=[]  NOutMax=[]  SumOutMin=[]  SumOutMax=[]  SaturationOutMin=[]  SaturationOutMax=[]  PParamMin=[]  PParamMax=[]  IParamMin=[]  IParamMax=[]  DParamMin=[]  DParamMax=[]  NParamMin=[]  NParamMax=[]  KbParamMin=[]  KbParamMax=[]  KtParamMin=[]  KtParamMax=[]  KbOutMin=[]  KbOutMax=[]  KtOutMin=[]  KtOutMax=[]  IntegratorOutMin=[]  IntegratorOutMax=[]  FilterOutMin=[]  FilterOutMax=[]  SumI1OutMin=[]  SumI1OutMax=[]  SumI2OutMin=[]  SumI2OutMax=[]  SumI3OutMin=[]  SumI3OutMax=[]  SumI4OutMin=[]  SumI4OutMax=[]  SumDOutMin=[]  SumDOutMax=[]  DifferentiatorOutMin=[]  DifferentiatorOutMax=[]  FilterDiffOutCoefMin=[]  FilterDiffOutCoefMax=[]  ReciprocalOutMin=[]  ReciprocalOutMax=[]  SumDenOutMin=[]  SumDenOutMax=[]  SumNumOutMin=[]  SumNumOutMax=[]  DivideOutMin=[]  DivideOutMax=[]  UdiffTsProdOutMin=[]  UdiffTsProdOutMax=[]  NTsProdOutMin=[]  NTsProdOutMax=[]  UintegralTsProdOutMin=[]  UintegralTsProdOutMax=[]  UngainTsProdOutMin=[]  UngainTsProdOutMax=[]  ClampingZeroOutDataTypeStr=Inherit: Inherit via back propagation  ClampingZeroOutMin=[]  ClampingZeroOutMax=[]  FilterDenConstantOutDataTypeStr=Inherit: Inherit via back propagation  FilterDenConstantOutMin=[]  FilterDenConstantOutMax=[]  PCopyOutDataTypeStr=Inherit: Inherit via back propagation  PCopyOutMin=[]  PCopyOutMax=[]  NCopyOutDataTypeStr=Inherit: Inherit via back propagation  NCopyOutMin=[]  NCopyOutMax=[]  IntegratorContinuousStateAttributes=''  IntegratorStateMustResolveToSignalObject=off  IntegratorRTWStateStorageClass=Auto  FilterContinuousStateAttributes=''  FilterStateMustResolveToSignalObject=off  FilterRTWStateStorageClass=Auto  ParallelPVariant=InternalParameters  IdealPVariant=Disabled  IVariant=InternalParameters  DVariant=InternalParameters  IntegratorVariant=Continuous  SatVariant=Disabled  AWVariant=Passthrough  PCopyVariant=Disabled  TRVariant=Disabled  FdbkBlocksVariant=Forward  IdealPFdbkVariant=Disabled  SatFdbkVariant=Disabled  DerivativeFilterVariant=ContFilter  NVariant=InternalParameters  NCopyVariant=Disabled  FilterICVariant=InternalICsFilter  IntegratorICVariant=InternalICs  ExternalResetVariant=Disabled  TRSumVariant=Passthrough  SumFdbkVariant=Disabled  SumVariant=Sum_PID  TsampFilterVariant=InternalTs  TsampNgainVariant=Passthrough  TsampIntegralVariant=Disabled_SignalSpec  ExternalSaturationOutDataTypeStr=Inherit: Same as second input  DerivativeSourceVariant=ErrorSignal  PreIntVariant=InternalPreInt
  Saturation{1..4} (4 alike) : Saturate  UpperLimit=25  LowerLimit=-25
  Scope1 : Scope  NumInputPorts=4
      settings: ActiveDisplayYMinimum=-6.8032570535996717  ActiveDisplayYMaximum=1.8406276967016679  DataLoggingVariableName=ScopeData14
  Scope2 : Scope  NumInputPorts=4
      settings: ActiveDisplayYMinimum=-2.9013447972961286  ActiveDisplayYMaximum=0.69036785474813156  DataLoggingVariableName=ScopeData9
  Sum{,1,6,11} (4 alike) : Sum  Inputs=++|
  Sum{2..5} (4 alike) : Sum  Inputs=+-|
  Transfer Fcn{1..4} (4 alike) : TransferFcn  Numerator=[1024]  Denominator="[1  25.6 1024]"
  Torque_wheels : Outport
  tag scope: error_vels=global
  wires:
  Transfer Fcn2/1 -> Saturation1/1
  Sum3/1 -> PID Controller4/1, Mux1/2
  Demux2/2 -> Sum3/2
  Demux2/4 -> Sum5/2
  Transfer Fcn3/1 -> Saturation2/1
  Sum4/1 -> PID Controller3/1, Mux1/3
  Sum2/1 -> PID Controller2/1, Mux1/1
  feedback/1 -> Demux2/1
  Demux2/1 -> Sum2/2
  Transfer Fcn4/1 -> Saturation4/1
  Transfer Fcn1/1 -> Saturation3/1
  Sum5/1 -> Mux1/4, PID Controller1/1
  Demux2/3 -> Sum4/2
  Saturation2/1 -> Mux/3
  Saturation4/1 -> Mux/4
  Saturation3/1 -> Mux/2
  Saturation1/1 -> Mux/1
  Mux/1 -> Torque_wheels/1
  ref/1 -> Demux1/1
  Mux1/1 -> [error_vels]
  Demux1/4 -> Sum5/1, Scope2/4
  Demux1/3 -> Sum4/1, Scope2/3
  Demux1/2 -> Sum3/1, Scope2/2
  Demux1/1 -> Sum2/1, Scope2/1
  theta_error/1 -> Demux3/1
  PID Controller1/1 -> Sum11/2
  Demux3/1 -> Scope1/4, PID Controller5/1
  Demux3/2 -> PID Controller6/1, Scope1/3
  Demux3/3 -> PID Controller7/1, Scope1/2
  Demux3/4 -> Scope1/1, PID Controller8/1
  Sum1/1 -> Transfer Fcn2/1
  PID Controller2/1 -> Sum1/2
  PID Controller4/1 -> Sum6/2
  Sum6/1 -> Transfer Fcn1/1
  PID Controller3/1 -> Sum/2
  Sum/1 -> Transfer Fcn3/1
  Sum11/1 -> Transfer Fcn4/1
  PID Controller8/1 -> Gain2/1
  PID Controller6/1 -> Gain3/1
  PID Controller5/1 -> Gain1/1
  PID Controller7/1 -> Gain4/1
  Gain2/1 -> Sum1/1
  Gain4/1 -> Sum6/1
  Gain3/1 -> Sum/1
  Gain1/1 -> Sum11/1

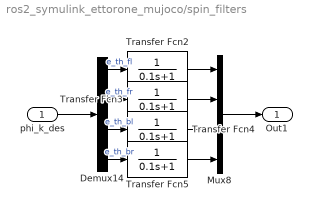
== system ros2_symulink_ettorone_mujoco/spin_filters ==
  phi_k_des : Inport
  Demux14 : Demux
  Mux8 : Mux
  Transfer Fcn{2..5} (4 alike) : TransferFcn  Denominator=[0.1 1]
  Out1 : Outport
  wires:
  Transfer Fcn4/1 -> Mux8/3
  Demux14/2 -> Transfer Fcn3/1  "e_th_fr"
  Transfer Fcn5/1 -> Mux8/4
  Mux8/1 -> Out1/1
  Transfer Fcn3/1 -> Mux8/2
  Demux14/3 -> Transfer Fcn4/1  "e_th_bl"
  Transfer Fcn2/1 -> Mux8/1
  Demux14/1 -> Transfer Fcn2/1  "e_th_fl"
  Demux14/4 -> Transfer Fcn5/1  "e_th_br"
  phi_k_des/1 -> Demux14/1

== matlab function ros2_symulink_ettorone_mujoco/ackermann_geometry ==
  data: v output; v_des input; phi_des input; phi output
function [v, phi] = fcn(v_des, phi_des)
% fcn robusta per 4WIS Ackermann-like
% evita NaN/Inf e discontinuità

% OUTPUT
phi = zeros(4,1);
v   = zeros(4,1);

% PARAMETRI
L = 0.64 ;
W = 0.50;
offset = 0.15;

% COSTANTI NUMERICHE
eps_phi = 1e-3;     % soglia angolo
eps_r   = 1e-6;     % per evitare divisioni per zero
eps_Ri  = 1e-3;     % raggio minimo ruota

% --------------------------------------------------
% GESTIONE SINGOLARITÀ (NO cot diretto per piccoli angoli)

if abs(phi_des) < eps_phi
    % moto rettilineo approssimato
    H = sign(phi_des + eps_phi) * 1e3;  % raggio molto grande
else
    H = (L/2) * cot(phi_des);
end

% --------------------------------------------------
% RAGGIO PRINCIPALE
R = sqrt((L/2)^2 + H^2);
R = max(R, eps_r);

% --------------------------------------------------
% ANGOLI DI STERZO (continui)
phi(1) = atan2( L*sin(phi_des),  L*cos(phi_des) - W*sin(phi_des) ); % FL
phi(2) = atan2( L*sin(phi_des),  L*cos(phi_des) + W*sin(phi_des) ); % FR

phi_des_b = -phi_des;

phi(3) = atan2( L*sin(phi_des_b), L*cos(phi_des_b) + W*sin(phi_des_b) ); % BL
phi(4) = atan2( L*sin(phi_des_b), L*cos(phi_des_b) - W*sin(phi_des_b) ); % BR

% --------------------------------------------------
% DISTANZE DAL CENTRO DI ROTAZIONE (ICR)

if H >= 0
    R_fl = sqrt((L/2)^2 + (H - W/2)^2) - offset;
    R_fr = sqrt((L/2)^2 + (H + W/2)^2) + offset;
    R_bl = sqrt((L/2)^2 + (H - W/2)^2) - offset;
    R_br = sqrt((L/2)^2 + (H + W/2)^2) + offset;
else
    R_fl = sqrt((L/2)^2 + (H - W/2)^2) + offset;
    R_fr = sqrt((L/2)^2 + (H + W/2)^2) - offset;
    R_bl = sqrt((L/2)^2 + (H - W/2)^2) + offset;
    R_br = sqrt((L/2)^2 + (H + W/2)^2) - offset;
end

% --------------------------------------------------
% EVITA RAGGI NEGATIVI O ZERO
R_fl = max(R_fl, eps_Ri);
R_fr = max(R_fr, eps_Ri);
R_bl = max(R_bl, eps_Ri);
R_br = max(R_br, eps_Ri);

% --------------------------------------------------
% VELOCITÀ RUOTE
v(1) = (R_fl / R) * v_des;
v(2) = (R_fr / R) * v_des;
v(3) = (R_bl / R) * v_des;
v(4) = (R_br / R) * v_des;

end

== matlab function ros2_symulink_ettorone_mujoco/control + motor torque linear dynamic (steering angles)/commentato ==
  data: u input; y output; v_centro input; v_ref input
function y = fcn(u, v_centro, v_ref)
%questo termine va a decadere se la velocita del centro del robot va ad
%allinearsi con la velocita delle ruote

% output
y = u *max(0,(1-v_centro/(v_ref + 1e-6)));


end

== matlab function ros2_symulink_ettorone_mujoco/control + motor torque linear dynamic (steering angles)/MATLAB Function1 ==
  data: u input; y output; v_centro input; v_ref input
function y = fcn(u, v_centro, v_ref)


% output
y = u *max(0,(1-v_centro/(v_ref + 1e-6)));


end

== matlab function ros2_symulink_ettorone_mujoco/control + motor torque linear dynamic (steering angles)/MATLAB Function2 ==
  data: u input; y output; v_centro input; v_ref input
function y = fcn(u, v_centro, v_ref)

% output
y = u *max(0,(1-v_centro/(v_ref + 1e-6)));


end

== matlab function ros2_symulink_ettorone_mujoco/Crab steering ==
  data: v output; v_des input; phi_des input; phi output
function [v,phi] = fcn(v_des, phi_des)
% fcn  calcola angoli di sterzo e velocità ruote per 4WIS secondo la
% geometria di ackerman
%
%   phi_des : direzione desiderata (rad)
%   V_des   : velocità desiderata al CG (m/s)
%   L       : passo longitudinale CG→asse anteriore (m)
%   W       : semicarreggiata (m)


phi = zeros(4,1);
v   = zeros(4,1);
enable = 2;
if enable == 2
    if abs(phi_des) >= pi/3
        phi_des = pi/3;
    end
    v(1) = v_des;
    v(2) = v_des;
    v(3) = v_des;
    v(4) = v_des;

    phi(1) = phi_des;
    phi(2) = phi_des;
    phi(3) = phi_des;
    phi(4) = phi_des;

end

== matlab function ros2_symulink_ettorone_mujoco/spin mod ==
  data: v output; v_des input; phi output
function [v, phi] = fcn(v_des)% geometria di ackerman
%
%   phi_des : direzione desiderata (rad)
%   V_des   : velocità desiderata al CG (m/s)
%   L       : passo longitudinale CG→asse anteriore (m)
%   W       : semicarreggiata (m)

phi = zeros(4,1);
v   = zeros(4,1);
alpha = 0.668;
v(1) = v_des;
v(2) = -v_des;
v(3) = v_des;
v(4) = -v_des;

phi(1) = -alpha;
phi(2) = alpha;
phi(3) = phi(2);
phi(4) = phi(1);

== matlab function ros2_symulink_ettorone_mujoco/control + motor torque linear dynamic (steering angles)/MATLAB Function3 ==
  data: u input; y output; v_centro input; v_ref input
function y = fcn(u, v_centro, v_ref)


% output
y = u *max(0,(1-v_centro/(v_ref + 1e-6)));

end
